simulink model "sampleModel1450"  (R2023a)
settings: Solver=VariableStepAuto  StartTime=0.0  StopTime=10.0  RelTol=1e-3
libraries: hdlsllib x2, simulink x1
settings Model: Creator=user1  LastModifiedBy=user1

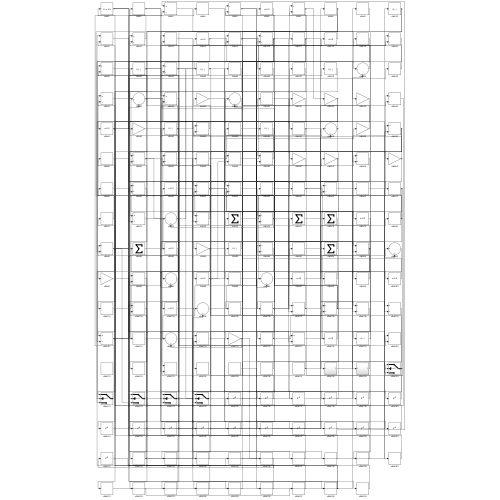
[thumbnail: Simulink's stored preview of the top-level diagram]
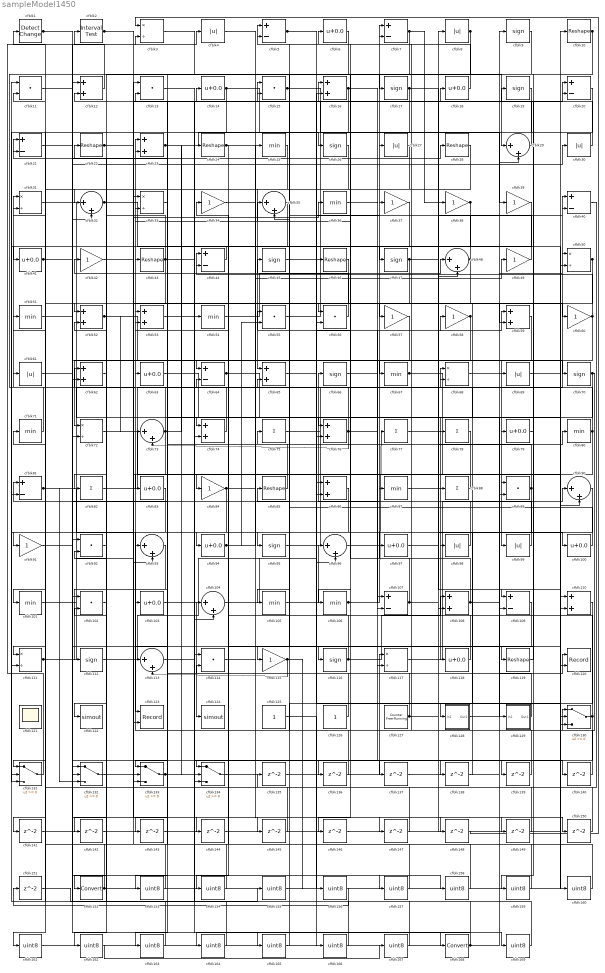
== system sampleModel1450 ==
  cfblk1 : simulink/Logic and Bit Operations/Detect Change  vinit=0  OutDataTypeStr=boolean
      settings: LibrarySourceBlock=|
      | hdlsllib/Logic and Bit
      | Operations/Detect
      | Change
  cfblk{10,22,24,28,43,46,85,119} (8 alike) : Reshape
  cfblk{6,14,18,41,63,79,83,94,97,100,103,118} (12 alike) : Bias  Bias=0.0  SaturateOnIntegerOverflow=off
  cfblk{25,36,51,54,67,71,80,87,101,105..106} (11 alike) : MinMax
  cfblk{11,13,15,55..56,89,92,102,114} (9 alike) : DotProduct  OutDataTypeStr=Inherit: Inherit via internal rule
  cfblk{29,32,35,48,73,90,93,96,104,113} (10 alike) : Sum  Inputs=|++
  cfblk{5,7,20..21,40,44,64,81,107,109} (10 alike) : Sum  Inputs=+-
  cfblk{12,16,23,52..53,59,62,65,74,76,86,108,110} (13 alike) : Sum
  cfblk{3,31,33,50,68,72,111,117} (8 alike) : Product  Inputs=*/  RndMeth=Zero  SaturateOnIntegerOverflow=on
  cfblk{9,17,19,26,45,47,66,70,95,112,116} (11 alike) : Signum
  cfblk{34,37..39,42,49,57..58,60,84,91,115} (12 alike) : Gain
  cfblk120 : Record  FileSettingsInternal="{\"entries\":[{\"content\":{\"excelSettings\":{\"content\":{},\"type\":\"Streamout.ExcelSettings\"}},\"type\":\"Streamout.FileSettingStorage\",\"uuid\":\"\"}],\"packageUris\":[\"http:\\/\\/schema.mathworks.com\\/mf0\\/streamout_blocks\\/R2020a\"],\"version\":\"1.0\"}"  Layout=[1 1]  SignalsInternal="{\"entries\":[{\"content\":{},\"type\":\"RecordBlkView.InputSignals\",\"uuid\":\"\"}],\"packageUris\":[\"http:\\/\\/schema.mathworks.com\\/mf0\\/streamout_blocks\\/R2020a\"],\"version\":\"1.0\"}"  VisualizationBindings="{\"xyplotplugin\":{\"info\":[{\"series\":[{\"bindingParametersList\":[{\"parameter\":\"X-Axis\",\"signalID\":755,\"signalName\":\"cfblk128\"},{\"parameter\":\"Y-Axis\",\"signalID\":760,\"signalName\":\"cfblk1\"}],\"seriesID\":12178}],\"subplotID\":1}]}}"  CompatibilityTag=XY  st=-1
  cfblk121 : Scope
      settings: Floating=on
  cfblk122 : ToWorkspace  VariableName=simout  SaveFormat=Timeseries  SampleTime=-1
  cfblk123 : Record  FileSettingsInternal="{\"entries\":[{\"content\":{\"excelSettings\":{\"content\":{},\"type\":\"Streamout.ExcelSettings\"}},\"type\":\"Streamout.FileSettingStorage\",\"uuid\":\"\"}],\"packageUris\":[\"http:\\/\\/schema.mathworks.com\\/mf0\\/streamout_blocks\\/R2020a\"],\"version\":\"1.0\"}"  Layout=[1 1]  SignalsInternal="{\"entries\":[{\"content\":{},\"type\":\"RecordBlkView.InputSignals\",\"uuid\":\"\"}],\"packageUris\":[\"http:\\/\\/schema.mathworks.com\\/mf0\\/streamout_blocks\\/R2020a\"],\"version\":\"1.0\"}"  VisualizationBindings="{\"xyplotplugin\":{\"info\":[{\"series\":[{\"bindingParametersList\":[{\"parameter\":\"X-Axis\",\"signalID\":764,\"signalName\":\"cfblk83\"},{\"parameter\":\"Y-Axis\",\"signalID\":768,\"signalName\":\"cfblk8\"}],\"seriesID\":30120}],\"subplotID\":1}]}}"  CompatibilityTag=XY  st=-1
  cfblk124 : ToWorkspace  VariableName=simout  SaveFormat=Timeseries  SampleTime=-1
  cfblk125 : Constant  SampleTime=-1
  cfblk126 : Constant  SampleTime=-1
  cfblk127 : hdlsllib/Sources/Counter Free-Running  NumBits=16  tsamp=-1
  cfblk128 : Subsystem
      settings: LibrarySourceBlock=|
      | hdlsllib/Ports &
      | Subsystems/Subsystem
  cfblk129 : Subsystem
      settings: LibrarySourceBlock=|
      | hdlsllib/Ports &
      | Subsystems/Subsystem
  cfblk{130..134} (5 alike) : Switch  SaturateOnIntegerOverflow=off  InputSameDT=off
  cfblk{135..151} (17 alike) : Delay  SampleTime=1
  cfblk152 : DataTypeConversion  SaturateOnIntegerOverflow=off  RndMeth=Floor
  cfblk{153..167,169} (16 alike) : DataTypeConversion  OutDataTypeStr=uint8  SaturateOnIntegerOverflow=off  RndMeth=Floor
  cfblk168 : DataTypeConversion  SaturateOnIntegerOverflow=off  RndMeth=Floor
  cfblk2 : hdlsllib/Logic and Bit Operations/Interval Test  IntervalClosedRight=on  uplimit=0.5  IntervalClosedLeft=on  lowlimit=-0.5  OutDataTypeStr=boolean
  cfblk{4,8,27,30,61,69,98..99} (8 alike) : Abs  SaturateOnIntegerOverflow=off
  cfblk{75,77..78,82,88} (5 alike) : Sum  Inputs=+
  wires:
  cfblk110/1 -> cfblk23/1
  cfblk83/1 -> cfblk123/1
  cfblk111/1 -> cfblk63/1, cfblk87/1, cfblk32/2
  cfblk99/1 -> cfblk66/1
  cfblk52/1 -> cfblk99/1, cfblk73/1
  cfblk26/1 -> cfblk65/1
  cfblk65/1 -> cfblk58/1
  cfblk130/1 -> cfblk53/1, cfblk134/3
  cfblk117/1 -> cfblk90/1
  cfblk71/1 -> cfblk29/1
  cfblk80/1 -> cfblk23/2, cfblk107/2, cfblk64/2
  cfblk107/1 -> cfblk7/1, cfblk109/1
  cfblk84/1 -> cfblk25/1, cfblk142/1
  cfblk43/1 -> cfblk21/2, cfblk47/1, cfblk153/1, cfblk161/1
  cfblk73/1 -> cfblk31/1, cfblk113/1, cfblk133/2, cfblk24/1
  cfblk55/1 -> cfblk18/1
  cfblk98/1 -> cfblk6/1
  cfblk77/1 -> cfblk118/1
  cfblk48/1 -> cfblk93/1, cfblk12/2
  cfblk29/1 -> cfblk14/1
  cfblk22/1 -> cfblk20/1, cfblk57/1
  cfblk46/1 -> cfblk56/1
  cfblk95/1 -> cfblk68/1
  cfblk131/1 -> cfblk4/1
  cfblk57/1 -> cfblk72/1
  cfblk18/1 -> cfblk5/1
  cfblk20/1 -> cfblk95/1
  cfblk87/1 -> cfblk98/1
  cfblk85/1 -> cfblk75/1
  cfblk106/1 -> cfblk77/1, cfblk59/1
  cfblk23/1 -> cfblk26/1, cfblk134/2
  cfblk116/1 -> cfblk108/1, cfblk65/2
  cfblk75/1 -> cfblk27/1
  cfblk127/1 -> cfblk43/1, cfblk80/1
  cfblk49/1 -> cfblk15/1
  cfblk105/1 -> cfblk96/1
  cfblk6/1 -> cfblk103/1
  cfblk103/1 -> cfblk124/1
  cfblk30/1 -> cfblk16/1
  cfblk92/1 -> cfblk152/1
  cfblk37/1 -> cfblk72/2
  cfblk31/1 -> cfblk129/1(In1)
  cfblk51/1 -> cfblk168/1
  cfblk56/1 -> cfblk42/1
  cfblk60/1 -> cfblk44/1, cfblk133/1
  cfblk101/1 -> cfblk36/1
  cfblk54/1 -> cfblk48/1
  cfblk72/1 -> cfblk88/1
  cfblk2/1 -> cfblk33/1, cfblk144/1
  cfblk35/1 -> cfblk101/1
  cfblk82/1 -> cfblk40/1
  cfblk134/1 -> cfblk117/1
  cfblk67/1 -> cfblk90/2, cfblk40/2
  cfblk68/1 -> cfblk9/1
  cfblk133/1 -> cfblk15/2, cfblk148/1
  cfblk81/1 -> cfblk93/2, cfblk117/2, cfblk3/2, cfblk132/3
  cfblk104/1 -> cfblk20/2
  cfblk16/1 -> cfblk35/2, cfblk81/2, cfblk59/2, cfblk86/2
  cfblk108/1 -> cfblk55/1, cfblk62/1, cfblk50/1, cfblk33/2
  cfblk38/1 -> cfblk131/1, cfblk131/3
  cfblk44/1 -> cfblk41/1
  cfblk1/1 -> cfblk67/1, cfblk120/2, cfblk158/1
  cfblk118/1 -> cfblk53/2
  cfblk93/1 -> cfblk112/1
  cfblk14/1 -> cfblk46/1, cfblk32/1
  cfblk126/1 -> cfblk34/1
  cfblk76/1 -> cfblk22/1, cfblk89/2, cfblk73/2
  cfblk12/1 -> cfblk2/1
  cfblk15/1 -> cfblk39/1, cfblk130/3
  cfblk66/1 -> cfblk97/1
  cfblk3/1 -> cfblk17/1
  cfblk79/1 -> cfblk119/1
  cfblk62/1 -> cfblk122/1
  cfblk10/1 -> cfblk115/1, cfblk159/1
  cfblk115/1 -> cfblk113/2, cfblk156/1
  cfblk109/1 -> cfblk134/1
  cfblk74/1 -> cfblk61/1
  cfblk9/1 -> cfblk116/1
  cfblk89/1 -> cfblk21/1, cfblk128/1(In1), cfblk131/2
  cfblk78/1 -> cfblk84/1
  cfblk47/1 -> cfblk105/1, cfblk100/1
  cfblk28/1 -> cfblk76/1
  cfblk24/1 -> cfblk74/1, cfblk150/1
  cfblk5/1 -> cfblk70/1, cfblk89/1
  cfblk86/1 -> cfblk94/1
  cfblk7/1 -> cfblk52/1, cfblk38/1
  cfblk42/1 -> cfblk60/1
  cfblk17/1 -> cfblk111/1, cfblk110/2, cfblk62/2
  cfblk70/1 -> cfblk130/1, cfblk163/1
  cfblk112/1 -> cfblk37/1
  cfblk19/1 -> cfblk111/2
  cfblk58/1 -> cfblk106/1, cfblk133/3
  cfblk59/1 -> cfblk74/2
  cfblk8/1 -> cfblk82/1, cfblk123/2
  cfblk119/1 -> cfblk19/1
  cfblk36/1 -> cfblk107/1
  cfblk88/1 -> cfblk83/1
  cfblk32/1 -> cfblk104/1, cfblk110/1
  cfblk63/1 -> cfblk130/2
  cfblk97/1 -> cfblk8/1
  cfblk34/1 -> cfblk76/2
  cfblk21/1 -> cfblk64/1
  cfblk27/1 -> cfblk91/1
  cfblk41/1 -> cfblk30/1, cfblk28/1
  cfblk64/1 -> cfblk96/2, cfblk109/2
  cfblk45/1 -> cfblk79/1
  cfblk50/1 -> cfblk78/1, cfblk132/2, cfblk154/1
  cfblk94/1 -> cfblk49/1, cfblk55/2
  cfblk100/1 -> cfblk45/1
  cfblk128/1(Out1) -> cfblk120/1
  cfblk129/1(Out1) -> cfblk81/1
  cfblk40/1 -> cfblk135/1
  cfblk135/1 -> cfblk56/2
  cfblk90/1 -> cfblk136/1
  cfblk136/1 -> cfblk44/2
  cfblk53/1 -> cfblk137/1
  cfblk137/1 -> cfblk29/2
  cfblk91/1 -> cfblk138/1
  cfblk138/1 -> cfblk68/2
  cfblk96/1 -> cfblk139/1
  cfblk139/1 -> cfblk5/2
  cfblk4/1 -> cfblk140/1
  cfblk140/1 -> cfblk7/2
  cfblk25/1 -> cfblk141/1
  cfblk141/1 -> cfblk16/2
  cfblk142/1 -> cfblk104/2
  cfblk33/1 -> cfblk143/1
  cfblk143/1 -> cfblk48/2
  cfblk144/1 -> cfblk50/2
  cfblk132/1 -> cfblk145/1
  cfblk145/1 -> cfblk52/2
  cfblk39/1 -> cfblk146/1
  cfblk146/1 -> cfblk108/2
  cfblk61/1 -> cfblk147/1
  cfblk147/1 -> cfblk31/2
  cfblk148/1 -> cfblk3/1
  cfblk114/1 -> cfblk149/1
  cfblk149/1 -> cfblk35/1
  cfblk150/1 -> cfblk1/1
  cfblk152/1 -> cfblk86/1, cfblk132/1, cfblk54/1
  cfblk153/1 -> cfblk92/1
  cfblk154/1 -> cfblk92/2
  cfblk151/1 -> cfblk155/1
  cfblk155/1 -> cfblk10/1
  cfblk156/1 -> cfblk151/1
  cfblk13/1 -> cfblk157/1
  cfblk157/1 -> cfblk71/1
  cfblk158/1 -> cfblk13/1
  cfblk159/1 -> cfblk13/2
  cfblk69/1 -> cfblk160/1
  cfblk160/1 -> cfblk114/2
  cfblk161/1 -> cfblk69/1
  cfblk102/1 -> cfblk162/1
  cfblk163/1 -> cfblk102/1
  cfblk164/1 -> cfblk102/2
  cfblk11/1 -> cfblk165/1
  cfblk165/1 -> cfblk85/1
  cfblk125/1 -> cfblk166/1
  cfblk166/1 -> cfblk11/1
  cfblk162/1 -> cfblk167/1
  cfblk167/1 -> cfblk11/2
  cfblk168/1 -> cfblk164/1, cfblk12/1, cfblk114/1
  cfblk113/1 -> cfblk169/1
  cfblk169/1 -> cfblk51/1

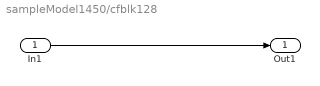
== system sampleModel1450/cfblk128 ==
  In1 : Inport
  Out1 : Outport
  wires:
  In1/1 -> Out1/1

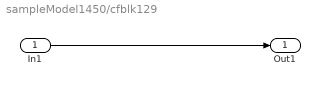
== system sampleModel1450/cfblk129 ==
  In1 : Inport
  Out1 : Outport
  wires:
  In1/1 -> Out1/1
